simulink model "Model1"  (R2014b)
settings: Solver=ode45  StartTime=0.0  StopTime=100.0  RelTol=1e-4
values from neighbouring files (symbols this model uses):
  A = [-1 Sr1 1 0 0 0; 0 -1 0 1 0 0; -1 Sr2 0 0 1 0; 0 -1 0 0 0 1]    [Internalforce_symbolic.m]    (also in Model1Init.m = [-eye(3),eye(3),zeros(3);-eye(3),zeros(3),eye(3)])
  d1 = 5    [Model1Init.m]
  d2 = 5    [Model1Init.m]
  G_Mplus = [m1/m0 *eye(3);m2/m0 *eye(3)]    [Model1Init.m]
  k1 = 1    [Model1Init.m]
  k2 = 1    [Model1Init.m]
  m0 = 20    [Model1Init.m]
  m1 = 10    [Model1Init.m]
  m2 = 10    [Model1Init.m]
libraries: dspinverses x1
settings Model: Creator=Martin  LastModifiedBy=Martin

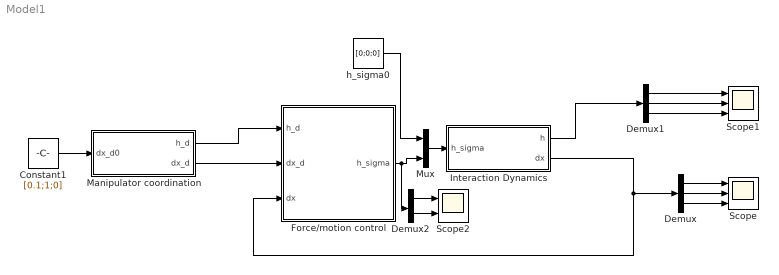
== system Model1 ==
  Constant1 : Constant  Value=[0.1;1;0]
  Demux : Demux  Outputs=3
  Demux1 : Demux  Outputs=3
  Demux2 : Demux  Outputs=2
  Force/motion control : Subsystem
  Interaction Dynamics : Subsystem
  Manipulator coordination : Subsystem
  Mux : Mux  Inputs=2
  Scope : Scope  NumInputPorts=3
      settings: ShowLegends=on  YMin=-5~-5~-5  YMax=5~5~5
  Scope1 : Scope  NumInputPorts=3
      settings: ShowLegends=on  YMin=-5~-5~-5  YMax=5~5~5
  Scope2 : Scope  NumInputPorts=2
      settings: ShowLegends=on  YMin=-5~-5  YMax=5~5  SaveName=ScopeData2
  h_sigma0 : Constant  Value=[0;0;0]
  wires:
  Interaction Dynamics/2(dx) -> Force/motion control/3(dx), Demux/1
  Demux/1 -> Scope/1
  Demux/2 -> Scope/2
  Demux/3 -> Scope/3
  Mux/1 -> Interaction Dynamics/1(h_sigma)
  Force/motion control/1(h_sigma) -> Demux2/1, Mux/2
  h_sigma0/1 -> Mux/1
  Manipulator coordination/2(dx_d) -> Force/motion control/2(dx_d)
  Manipulator coordination/1(h_d) -> Force/motion control/1(h_d)
  Constant1/1 -> Manipulator coordination/1(dx_d0)
  Interaction Dynamics/1(h) -> Demux1/1
  Demux1/1 -> Scope1/1
  Demux1/2 -> Scope1/2
  Demux1/3 -> Scope1/3
  Demux2/2 -> Scope2/2
  Demux2/1 -> Scope2/1

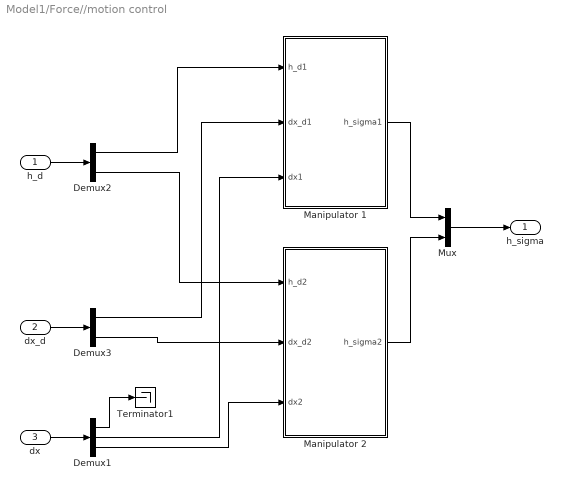
== system Model1/Force//motion control ==
  h_d : Inport
  dx_d : Inport  Port=2
  dx : Inport  Port=3
  Demux1 : Demux  Outputs=3
  Demux2 : Demux  Outputs=2
  Demux3 : Demux  Outputs=2
  Manipulator 1 : Subsystem
  Manipulator 2 : Subsystem
  Mux : Mux  Inputs=2
  Terminator1 : Terminator
  h_sigma : Outport
  wires:
  Manipulator 1/1(h_sigma1) -> Mux/1
  Manipulator 2/1(h_sigma2) -> Mux/2
  Mux/1 -> h_sigma/1
  Demux1/3 -> Manipulator 2/3(dx2)
  Demux1/2 -> Manipulator 1/3(dx1)
  Demux1/1 -> Terminator1/1
  dx_d/1 -> Demux3/1
  h_d/1 -> Demux2/1
  Demux2/1 -> Manipulator 1/1(h_d1)
  Demux2/2 -> Manipulator 2/1(h_d2)
  Demux3/1 -> Manipulator 1/2(dx_d1)
  Demux3/2 -> Manipulator 2/2(dx_d2)
  dx/1 -> Demux1/1

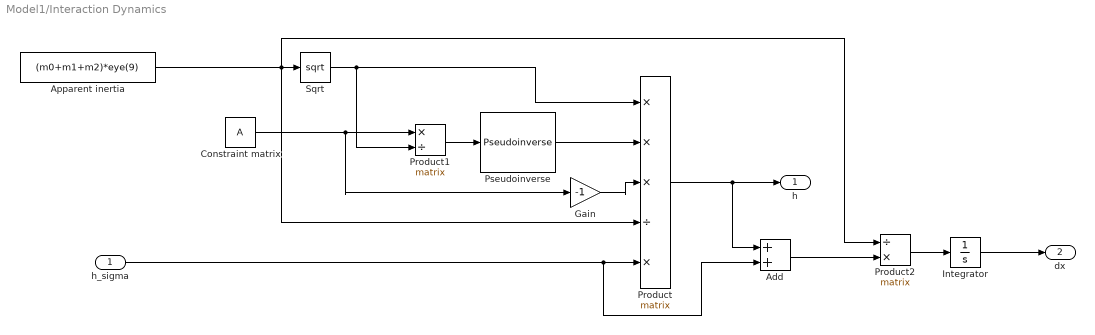
== system Model1/Interaction Dynamics ==
  h_sigma : Inport
  Add : Sum
  Apparent inertia : Constant  Value=(m0+m1+m2)*eye(9)
  Constraint matrix : Constant  Value=A
  Gain : Gain  Gain=-1
  Integrator : Integrator
  Product : Product  Inputs=***/*  Multiplication=Matrix(*)
  Product1 : Product  Inputs=*/  Multiplication=Matrix(*)
  Product2 : Product  Inputs=/*  Multiplication=Matrix(*)
  Pseudoinverse : dspinverses/Pseudoinverse  wanterr=off
  Sqrt : Sqrt  SaturateOnIntegerOverflow=on
  h : Outport
  dx : Outport  Port=2
  wires:
  Sqrt/1 -> Product1/2, Product/1
  Pseudoinverse/1 -> Product/2
  Product1/1 -> Pseudoinverse/1
  Constraint matrix/1 -> Gain/1, Product1/1
  h_sigma/1 -> Add/2, Product/5
  Product2/1 -> Integrator/1
  Integrator/1 -> dx/1
  Apparent inertia/1 -> Product2/1, Product/4, Sqrt/1
  Product/1 -> Add/1, h/1
  Gain/1 -> Product/3
  Add/1 -> Product2/2

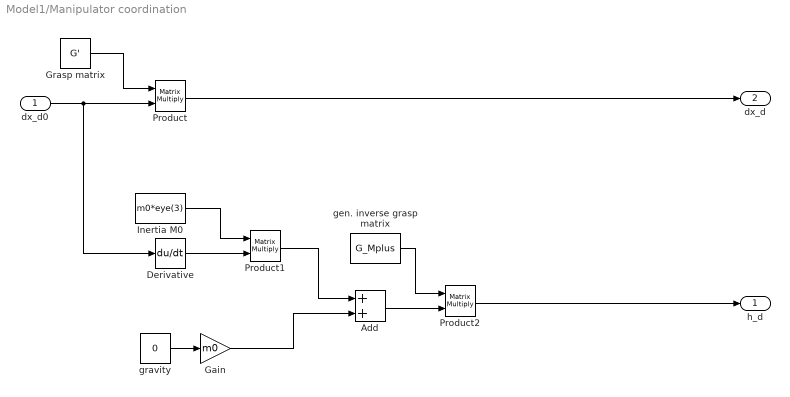
== system Model1/Manipulator coordination ==
  dx_d0 : Inport
  Add : Sum
  Derivative : Derivative
  Gain : Gain  Gain=m0
  Grasp matrix : Constant  Value=G'
  Inertia M0 : Constant  Value=m0*eye(3)
  Product : Product  Multiplication=Matrix(*)
  Product1 : Product  Multiplication=Matrix(*)
  Product2 : Product  Multiplication=Matrix(*)
  gen. inverse grasp matrix : Constant  Value=G_Mplus
  gravity : Constant  Value=0
  h_d : Outport
  dx_d : Outport  Port=2
  wires:
  dx_d0/1 -> Derivative/1, Product/2
  Grasp matrix/1 -> Product/1
  Product/1 -> dx_d/1
  Derivative/1 -> Product1/2
  Inertia M0/1 -> Product1/1
  gravity/1 -> Gain/1
  Gain/1 -> Add/2
  Product1/1 -> Add/1
  Add/1 -> Product2/2
  gen. inverse grasp matrix/1 -> Product2/1
  Product2/1 -> h_d/1

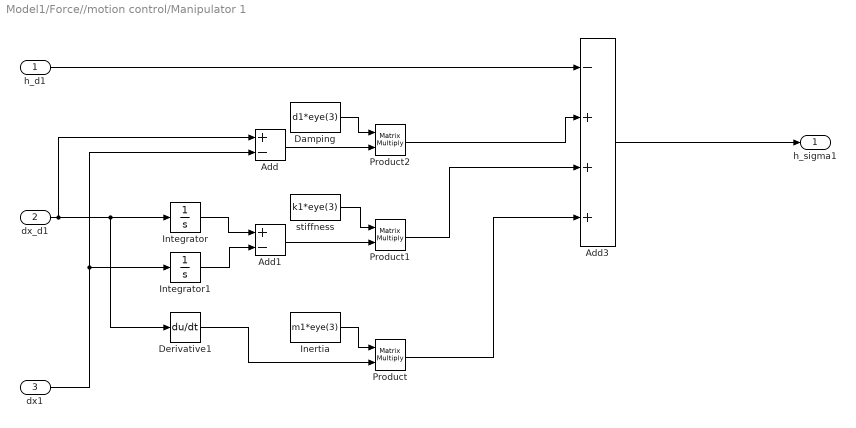
== system Model1/Force//motion control/Manipulator 1 ==
  h_d1 : Inport
  dx_d1 : Inport  Port=2
  dx1 : Inport  Port=3
  Add : Sum  Inputs=+-
  Add1 : Sum  Inputs=+-
  Add3 : Sum  Inputs=-+++
  Damping : Constant  Value=d1*eye(3)
  Derivative1 : Derivative
  Inertia : Constant  Value=m1*eye(3)
  Integrator : Integrator
  Integrator1 : Integrator
  Product : Product  Multiplication=Matrix(*)
  Product1 : Product  Multiplication=Matrix(*)
  Product2 : Product  Multiplication=Matrix(*)
  stiffness : Constant  Value=k1*eye(3)
  h_sigma1 : Outport
  wires:
  dx_d1/1 -> Add/1, Integrator/1, Derivative1/1
  dx1/1 -> Add/2, Integrator1/1
  Integrator1/1 -> Add1/2
  Integrator/1 -> Add1/1
  Derivative1/1 -> Product/2
  Add1/1 -> Product1/2
  Add/1 -> Product2/2
  Damping/1 -> Product2/1
  stiffness/1 -> Product1/1
  Inertia/1 -> Product/1
  Product/1 -> Add3/4
  Product1/1 -> Add3/3
  Product2/1 -> Add3/2
  h_d1/1 -> Add3/1
  Add3/1 -> h_sigma1/1

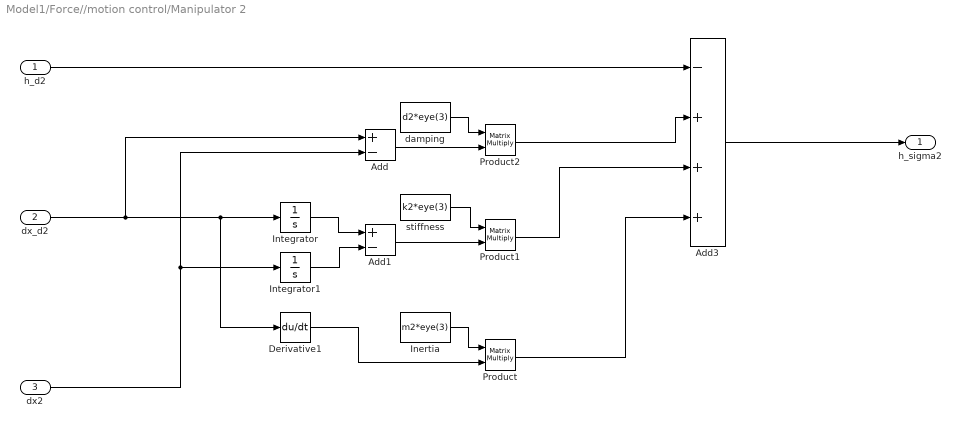
== system Model1/Force//motion control/Manipulator 2 ==
  h_d2 : Inport
  dx_d2 : Inport  Port=2
  dx2 : Inport  Port=3
  Add : Sum  Inputs=+-
  Add1 : Sum  Inputs=+-
  Add3 : Sum  Inputs=-+++
  Derivative1 : Derivative
  Inertia : Constant  Value=m2*eye(3)
  Integrator : Integrator
  Integrator1 : Integrator
  Product : Product  Multiplication=Matrix(*)
  Product1 : Product  Multiplication=Matrix(*)
  Product2 : Product  Multiplication=Matrix(*)
  damping : Constant  Value=d2*eye(3)
  stiffness : Constant  Value=k2*eye(3)
  h_sigma2 : Outport
  wires:
  dx_d2/1 -> Integrator/1, Derivative1/1, Add/1
  dx2/1 -> Integrator1/1, Add/2
  Integrator1/1 -> Add1/2
  Integrator/1 -> Add1/1
  Derivative1/1 -> Product/2
  Add1/1 -> Product1/2
  Add/1 -> Product2/2
  damping/1 -> Product2/1
  stiffness/1 -> Product1/1
  Inertia/1 -> Product/1
  Product/1 -> Add3/4
  Product1/1 -> Add3/3
  Product2/1 -> Add3/2
  h_d2/1 -> Add3/1
  Add3/1 -> h_sigma2/1
